simulink model "OfficalTeam58Code"  (R2023a)
settings: Solver=FixedStepAuto  StartTime=0.0  StopTime=inf  RelTol=1e-3  EnableMultiTasking=on
libraries: vexarmcortexlib x36, vexcommonlib x7, RoboticsPlayground x2
settings Model: Creator=arist  LastModifiedBy=arist
settings SolverCC: AutoInsertRateTranBlk=on
settings DataIOCC: LimitDataPoints=on  SignalLoggingSaveFormat=ModelDataLogs  ReturnWorkspaceOutputs=off
settings OptimizationCC: ExpressionDepthLimit=2147483647  LifeSpan=Inf  MaxStackSize=64  EfficientTunableParamExpr=on
settings DebuggingCC: UnderspecifiedInitializationDetection=Classic  MergeDetectMultiDrivingBlocksExec=none  InheritedTsInSrcMsg=none  MultiTaskRateTransMsg=warning  FcnCallInpInsideContextMsg=warning  StateNameClashWarn=warning  SFUnexpectedBacktrackingDiag=warning  SFNoUnconditionalDefaultTransitionDiag=warning  SFExecutionAtInitializationDiag=none  ArithmeticOperatorsInVariantConditions=warning
settings HardwareCC: ProdBitPerPointer=32  ProdBitPerSizeT=32  ProdBitPerPtrDiffT=32  ProdLargestAtomicInteger=Long  ProdLargestAtomicFloat=Double  ProdIntDivRoundTo=Undefined  ProdWordSize=32  ProdHWDeviceType=ARM Compatible->ARM Cortex
settings ModelReferenceCC: EnableRefExpFcnMdlSchedulingChecks=on  PropagateSignalLabelsOutOfModel=off
settings SFSimCC: MATLABDynamicMemAlloc=off  CustomCodeUndefinedFunction=UseInterfaceOnly
settings RTWCC: Description=Embedded Coder  SystemTargetFile=ert.tlc  HardwareBoard=ARM Cortex-based VEX Microcontroller  TemplateMakefile=ert_default_tmf  Toolchain=GNU Tools for VEX ARM Cortex
settings CodeAppCC: IgnoreCustomStorageClasses=off  CustomSymbolStrType=$N$R$M  StateflowObjectComments=on  InternalIdentifier=Classic
settings ERTTargetCC: CodeReplacementLibrary=GCC ARM Cortex-M3  MultiwordLength=2048  ConvertIfToSwitch=off  SuppressUnreachableDefaultCases=off

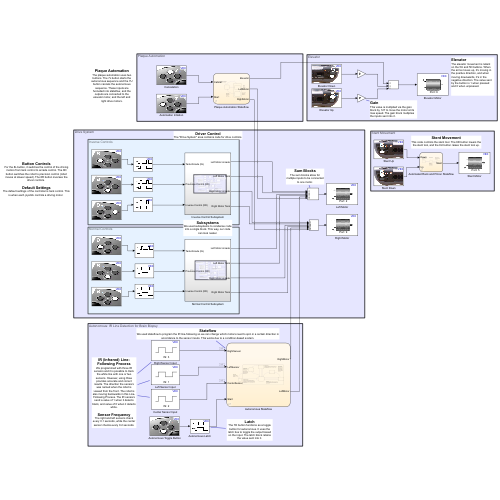
[thumbnail: Simulink's stored preview of the top-level diagram]
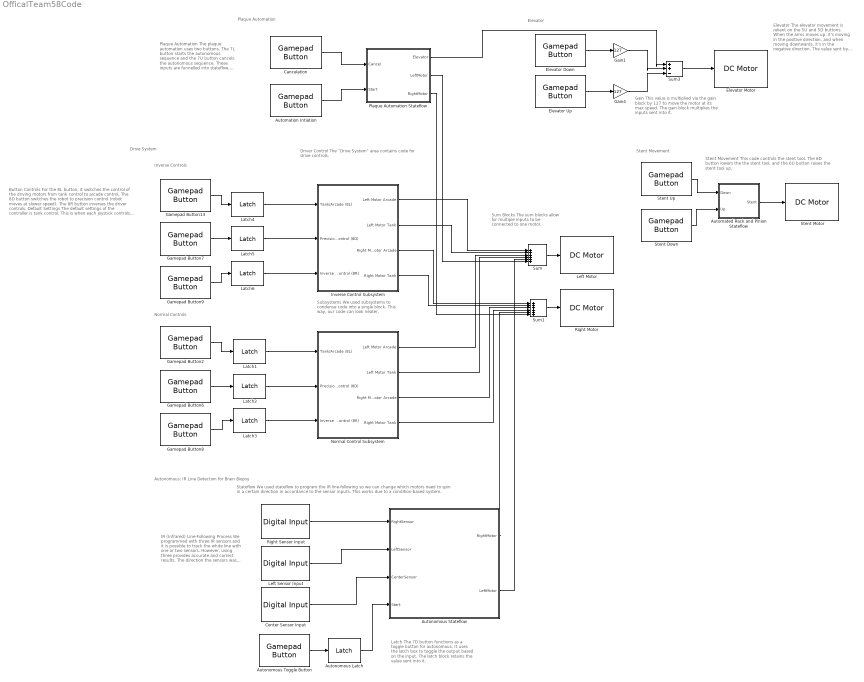
== system OfficalTeam58Code ==
  note: Driver Control
      | The "Drive System" area contains code for drive controls.
  note: Sum Blocks
      | The sum blocks allow for multiple inputs to be connected
      | to one motor.
  note: Subsystems
      | We used subsystems to condense code into a single block. This way, our code can look neater.
  note: Inverse Controls
  note: Autonomous: IR Line Detection for Brain Biopsy
  note: Drive System
  note: Normal Controls
  note: Plaque Automation
  note: Elevator
  note: Stent Movement
  note: Button Controls
      | For the 8L button, it switches the control of the driving motors from tank control to arcade control. The 8D button switches the robot to precision control (robot moves at slower speed). The 8R button inverses the driver controls.
      |
      | Default Settings
      | The default settings of the controller is tank control. This is when each joystick controls a driving motor.
  note: IR (Infrared) Line-Following Process
      | We programmed with three IR sensors and it is possible to track the white line with one or two sensors. However, using three provides accurate and correct results. The direction the sensors was named when the robot is viewed from the front. The robot is also moving backwards in this Line-Following Process. The IR sensors send a value of 1 when it detects black, and value of 0 when it detects white.
      |
      | Sensor Frequency
      | The right and left sensors check every 0.1 seconds, while the center sensor checks every 0.2 seconds.
  note: Latch
      | The 7D button functions as a toggle button for autonomous. It uses the latch box to toggle the output based on the input. The latch block retains the value sent into it.
  note: Stateflow
      | We used stateflow to program the IR line-following so we can change which motors need to spin in a certain direction in accordance to the sensor inputs. This works due to a condition-based system.
  note: Elevator
      | The elevator movement is reliant on the 5U and 5D buttons. When the arms moves up, it's moving in the positive direction, and when moving downwards, it's in the negative direction. The value sent by the button is 1 when pressed and 0 when unpressed.
  note: Plaque Automation
      | The plaque automation uses two buttons. The 7L button starts the autonomous sequence and the 7U button cancels the autonomous sequence. These inputs are funnelled into stateflow, and the outputs are connected to the elevator motor, and the left and right drive motors.
  note: Gain
      | This value is multiplied via the gain block by 127 to move the motor at its max speed. The gain block multiplies the inputs sent into it.
  note: Stent Movement
      | This code controls the stent tool. The 6D button lowers the the stent tool, and the 6U button raises the stent tool up.
  Automated Rack and Pinion Stateflow : Stateflow chart  AncestorBlock=RoboticsPlayground/Utilities and Hardware/Stateflow  TreatAsAtomicUnit=on
      settings: LibrarySourceBlock=RoboticsPlayground/Utilities and Hardware/Stateflow
  Automation Intiation : vexarmcortexlib/Gamepad/Gamepad Button  joystick=1  chan=7  button56=Down  button78=Left  SimulationIn=off  SampleTime=0.02
  Autonomous Latch : vexcommonlib/Latch  output0=off  BlockPlatform=vexv5
      settings: LibrarySourceBlock=vexv5lib/Utilities/Latch
  Autonomous Stateflow : Stateflow chart  AncestorBlock=RoboticsPlayground/Utilities and Hardware/Stateflow  TreatAsAtomicUnit=on
      settings: LibrarySourceBlock=RoboticsPlayground/Utilities and Hardware/Stateflow
  Autonomous Toggle Button : vexarmcortexlib/Gamepad/Gamepad Button  joystick=1  chan=7  button56=Up  button78=Down  SimulationIn=off  SampleTime=0.02
  Cancelation : vexarmcortexlib/Gamepad/Gamepad Button  joystick=1  chan=7  button56=Down  button78=Up  SimulationIn=off  SampleTime=0.02
  Center Sensor Input : vexarmcortexlib/Sensors/Digital Input  inChan=2  SimulationIn=off  SampleTime=0.2
  Elevator Down : vexarmcortexlib/Gamepad/Gamepad Button  joystick=1  chan=5  button56=Down  button78=Down  SimulationIn=off  SampleTime=0.02
  Elevator Motor : vexarmcortexlib/Actuators/DC Motor  motor=6  scaleFactor=1/13.5  SimulationOut=off
  Elevator Up : vexarmcortexlib/Gamepad/Gamepad Button  joystick=1  chan=5  button56=Up  button78=Down  SimulationIn=off  SampleTime=0.02
  Gain1 : Gain  Gain=127
  Gain4 : Gain  Gain=127
  Gamepad Button13 : vexarmcortexlib/Gamepad/Gamepad Button  joystick=1  chan=8  button56=Up  button78=Left  SimulationIn=off  SampleTime=0.02
  Gamepad Button2 : vexarmcortexlib/Gamepad/Gamepad Button  joystick=1  chan=8  button56=Up  button78=Left  SimulationIn=off  SampleTime=0.02
  Gamepad Button6 : vexarmcortexlib/Gamepad/Gamepad Button  joystick=1  chan=8  button56=Up  button78=Down  SimulationIn=off  SampleTime=0.02
  Gamepad Button7 : vexarmcortexlib/Gamepad/Gamepad Button  joystick=1  chan=8  button56=Up  button78=Down  SimulationIn=off  SampleTime=0.02
  Gamepad Button8 : vexarmcortexlib/Gamepad/Gamepad Button  joystick=1  chan=8  button56=Up  button78=Right  SimulationIn=off  SampleTime=0.02
  Gamepad Button9 : vexarmcortexlib/Gamepad/Gamepad Button  joystick=1  chan=8  button56=Up  button78=Right  SimulationIn=off  SampleTime=0.02
  Inverse Control Subsystem : Subsystem
  Latch{1..6} (6 alike) : vexcommonlib/Latch  output0=off  BlockPlatform=vexv5
      settings: LibrarySourceBlock=vexv5lib/Utilities/Latch
  Left Motor : vexarmcortexlib/Actuators/DC Motor  motor=2  scaleFactor=1/13.5  SimulationOut=off
  Left Sensor Input : vexarmcortexlib/Sensors/Digital Input  inChan=1  SimulationIn=off  SampleTime=0.1
  Normal Control Subsystem : Subsystem
  Plaque Automation Stateflow : Stateflow chart  AncestorBlock=RoboticsPlayground/Utilities and Hardware/Stateflow  TreatAsAtomicUnit=on
      settings: LibrarySourceBlock=RoboticsPlayground/Utilities and Hardware/Stateflow
  Right Motor : vexarmcortexlib/Actuators/DC Motor  motor=9  scaleFactor=1/13.5  SimulationOut=off
  Right Sensor Input : vexarmcortexlib/Sensors/Digital Input  inChan=3  SimulationIn=off  SampleTime=0.1
  Stent Down : vexarmcortexlib/Gamepad/Gamepad Button  joystick=1  chan=6  button56=Up  button78=Up  SimulationIn=off  SampleTime=0.02
  Stent Motor : vexarmcortexlib/Actuators/DC Motor  motor=5  scaleFactor=1/13.5  SimulationOut=off
  Stent Up : vexarmcortexlib/Gamepad/Gamepad Button  joystick=1  chan=6  button56=Down  button78=Left  SimulationIn=off  SampleTime=0.02
  Sum : Sum  Inputs=|++++++
  Sum1 : Sum  Inputs=|++++++
  Sum3 : Sum  Inputs=|++-
  wires:
  Gamepad Button2/1 -> Latch1/1
  Sum1/1 -> Right Motor/1
  Sum/1 -> Left Motor/1
  Autonomous Stateflow/1(RightMotor) -> Sum1/5
  Autonomous Stateflow/2(LeftMotor) -> Sum/5
  Autonomous Toggle Button/1 -> Autonomous Latch/1
  Center Sensor Input/1 -> Autonomous Stateflow/3(CenterSensor)
  Left Sensor Input/1 -> Autonomous Stateflow/2(LeftSensor)
  Right Sensor Input/1 -> Autonomous Stateflow/1(RightSensor)
  Gamepad Button6/1 -> Latch2/1
  Gamepad Button8/1 -> Latch3/1
  Latch1/1 -> Normal Control Subsystem/1(Tank/Arcade (8L))
  Latch2/1 -> Normal Control Subsystem/2(Precision Control (8D))
  Latch3/1 -> Normal Control Subsystem/3(Inverse Control (8R))
  Normal Control Subsystem/1(Left Motor Arcade) -> Sum/3
  Normal Control Subsystem/2(Left Motor Tank) -> Sum/4
  Normal Control Subsystem/3(Right Motor Arcade) -> Sum1/3
  Normal Control Subsystem/4(Right Motor Tank) -> Sum1/4
  Latch6/1 -> Inverse Control Subsystem/3(Inverse Control (8R))
  Latch5/1 -> Inverse Control Subsystem/2(Precision Control (8D))
  Gamepad Button9/1 -> Latch6/1
  Gamepad Button13/1 -> Latch4/1
  Gamepad Button7/1 -> Latch5/1
  Latch4/1 -> Inverse Control Subsystem/1(Tank/Arcade (8L))
  Inverse Control Subsystem/1(Left Motor Arcade) -> Sum/1
  Inverse Control Subsystem/2(Left Motor Tank) -> Sum/2
  Inverse Control Subsystem/4(Right Motor Tank) -> Sum1/2
  Inverse Control Subsystem/3(Right Motor Arcade) -> Sum1/1
  Autonomous Latch/1 -> Autonomous Stateflow/4(Start)
  Elevator Up/1 -> Gain4/1
  Plaque Automation Stateflow/2(LeftMotor) -> Sum/6
  Plaque Automation Stateflow/3(RightMotor) -> Sum1/6
  Gain1/1 -> Sum3/2
  Plaque Automation Stateflow/1(Elevator) -> Sum3/1
  Automation Intiation/1 -> Plaque Automation Stateflow/2(Start)
  Elevator Down/1 -> Gain1/1
  Cancelation/1 -> Plaque Automation Stateflow/1(Cancel)
  Sum3/1 -> Elevator Motor/1
  Gain4/1 -> Sum3/3
  Stent Up/1 -> Automated Rack and Pinion Stateflow/1(Down)
  Automated Rack and Pinion Stateflow/1(Stent) -> Stent Motor/1
  Stent Down/1 -> Automated Rack and Pinion Stateflow/2(Up)

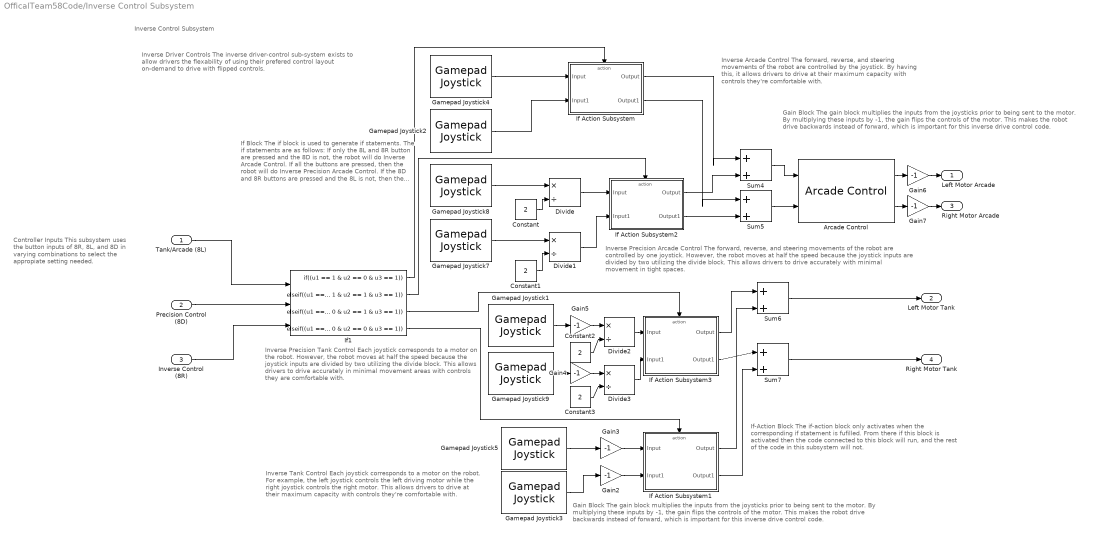
== system OfficalTeam58Code/Inverse Control Subsystem ==
  note: Inverse Driver Controls
      | The inverse driver-control sub-system exists to allow drivers
      | the flexability of using their prefered control layout on-demand to drive
      | with flipped controls.
  note: Inverse Control Subsystem
  note: If-Action Block
      | The if-action block only activates when the corresponding if statement is fufilled. From there if this block is activated then the code connected to this block will run, and the rest of the code in this subsystem will not.
  note: Controller Inputs
      | This subsystem uses the button inputs of 8R, 8L, and 8D
      | in varying combinations to select the appropiate setting needed.
  note: If Block
      | The if block is used to generate if statements. The if statements are as follows:
      | If only the 8L and 8R button are pressed and the 8D is not, the robot will do Inverse Arcade Control.
      | If all the buttons are pressed, then the robot will do Inverse Precision Arcade Control.
      | If the 8D and 8R buttons are pressed and the 8L is not, then the robot will do Inverse Precison Tank Control.
      | If only 8R is pressed and 8L and 8D are not, then the robot will do Inverse Tank Control.
  note: Inverse Precision Tank Control
      | Each joystick corresponds to a motor on the robot. However, the robot moves at half the speed because the joystick inputs are divided by two utilizing the divide block. This allows drivers to drive
      | accurately in minimal movement areas with controls they are
      | comfortable with.
  note: Inverse Tank Control
      | Each joystick corresponds to a motor on the robot. For example,
      | the left joystick controls the left driving motor while the right joystick
      | controls the right motor. This allows drivers to drive at their
      | maximum capacity with controls they're comfortable with.
  note: Inverse Precision Arcade Control
      | The forward, reverse, and steering movements of the robot are
      | controlled by one joystick. However, the robot moves at half the speed because the joystick inputs are divided by two utilizing the divide block. This allows drivers to drive accurately with minimal movement in tight spaces.
  note: Inverse Arcade Control
      | The forward, reverse, and steering movements of the robot are
      | controlled by the joystick. By having this, it allows drivers to
      | drive at their maximum capacity with controls they're comfortable
      | with.
  note: Gain Block
      | The gain block multiplies the inputs from the joysticks prior to being sent to the motor. By multiplying these inputs by -1, the gain flips the controls of the motor. This makes the robot drive backwards instead of forward, which is important for this inverse drive control code.
  note: Gain Block
      | The gain block multiplies the inputs from the joysticks prior to being sent to the motor. By multiplying these inputs by -1, the gain flips the controls of the motor. This makes the robot drive backwards instead of forward, which is important for this inverse drive control code.
  Tank/Arcade (8L) : Inport
  Precision Control (8D) : Inport  Port=2
  Inverse Control (8R) : Inport  Port=3
  Arcade Control : RoboticsPlayground/Utilities and Hardware/Arcade Control  SystemSampleTime=-1  VariantActivationTime=update diagram  Latency=0  AutoFrameSizeCalculation=off
      settings: SourceProductName=Robotics Playground
  Constant{,1..3} (4 alike) : Constant  Value=2
  Divide{,1..3} (4 alike) : Product  Inputs=*/
  Gain{2..7} (6 alike) : Gain  Gain=-1
  Gamepad Joystick{1,3..4,8} (4 alike) : vexarmcortexlib/Gamepad/Gamepad Joystick  joystick=1  chan=3  SimulationIn=off  SampleTime=0.02
  Gamepad Joystick2 : vexarmcortexlib/Gamepad/Gamepad Joystick  joystick=1  chan=4  SimulationIn=off  SampleTime=0.02
  Gamepad Joystick5 : vexarmcortexlib/Gamepad/Gamepad Joystick  joystick=1  chan=2  SimulationIn=off  SampleTime=0.02
  Gamepad Joystick7 : vexarmcortexlib/Gamepad/Gamepad Joystick  joystick=1  chan=4  SimulationIn=off  SampleTime=0.02
  Gamepad Joystick9 : vexarmcortexlib/Gamepad/Gamepad Joystick  joystick=1  chan=2  SimulationIn=off  SampleTime=0.02
  If Action Subsystem : Subsystem  TreatAsAtomicUnit=on
  If Action Subsystem1 : Subsystem  TreatAsAtomicUnit=on
  If Action Subsystem2 : Subsystem  TreatAsAtomicUnit=on
  If Action Subsystem3 : Subsystem  TreatAsAtomicUnit=on
  If1 : If  NumInputs=3  IfExpression=(u1 == 1 & u2 == 0 & u3 == 1)  ElseIfExpressions=(u1 == 1 & u2 == 1 & u3 == 1),(u1 == 0 & u2 == 1 & u3 == 1),(u1 == 0 & u2 == 0 & u3 == 1)  ShowElse=off
  Sum{4..7} (4 alike) : Sum  Inputs=|++
  Left Motor Arcade : Outport
  Left Motor Tank : Outport  Port=2
  Right Motor Arcade : Outport  Port=3
  Right Motor Tank : Outport  Port=4
  wires:
  Sum5/1 -> Arcade Control/2
  If1/4 -> If Action Subsystem1/Action
  If Action Subsystem1/1(Output) -> Sum6/2
  If1/3 -> If Action Subsystem3/Action
  If1/1 -> If Action Subsystem/Action
  If Action Subsystem2/1(Output) -> Sum4/2
  Divide2/1 -> If Action Subsystem3/1(Input)
  Constant1/1 -> Divide1/2
  If Action Subsystem1/2(Output1) -> Sum7/2
  Inverse Control (8R)/1 -> If1/3
  If Action Subsystem2/2(Output1) -> Sum5/2
  If Action Subsystem/2(Output1) -> Sum5/1
  Gamepad Joystick3/1 -> Gain2/1
  Sum6/1 -> Left Motor Tank/1
  If Action Subsystem/1(Output) -> Sum4/1
  Constant/1 -> Divide/2
  Divide1/1 -> If Action Subsystem2/2(Input1)
  If1/2 -> If Action Subsystem2/Action
  Divide3/1 -> If Action Subsystem3/2(Input1)
  Sum7/1 -> Right Motor Tank/1
  Constant3/1 -> Divide3/2
  Gamepad Joystick5/1 -> Gain3/1
  Sum4/1 -> Arcade Control/1
  Divide/1 -> If Action Subsystem2/1(Input)
  If Action Subsystem3/1(Output) -> Sum6/1
  Precision Control (8D)/1 -> If1/2
  Gamepad Joystick1/1 -> Gain5/1
  Gamepad Joystick9/1 -> Gain4/1
  Constant2/1 -> Divide2/2
  Arcade Control/1 -> Gain6/1
  If Action Subsystem3/2(Output1) -> Sum7/1
  Tank/Arcade (8L)/1 -> If1/1
  Arcade Control/2 -> Gain7/1
  Gamepad Joystick4/1 -> If Action Subsystem/1(Input)
  Gamepad Joystick8/1 -> Divide/1
  Gain2/1 -> If Action Subsystem1/2(Input1)
  Gain3/1 -> If Action Subsystem1/1(Input)
  Gain5/1 -> Divide2/1
  Gain4/1 -> Divide3/1
  Gamepad Joystick2/1 -> If Action Subsystem/2(Input1)
  Gamepad Joystick7/1 -> Divide1/1
  Gain6/1 -> Left Motor Arcade/1
  Gain7/1 -> Right Motor Arcade/1

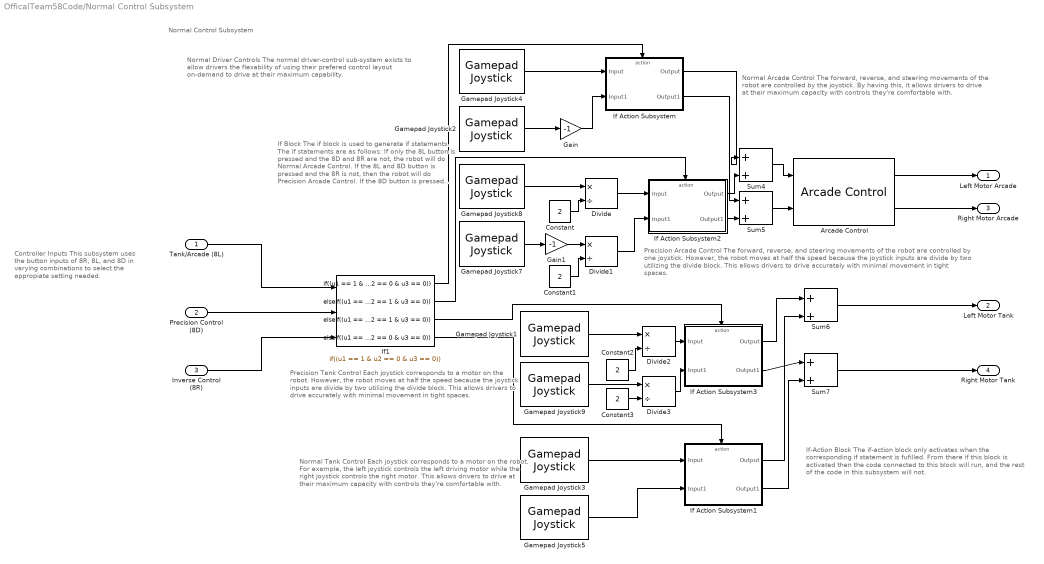
== system OfficalTeam58Code/Normal Control Subsystem ==
  note: If-Action Block
      | The if-action block only activates when the corresponding if statement is fufilled. From there if this block is activated then the code connected to this block will run, and the rest of the code in this subsystem will not.
  note: If Block
      | The if block is used to generate if statements. The if statements are as follows:
      | If only the 8L button is pressed and the 8D and 8R are not, the robot will do Normal Arcade Control.
      | If the 8L and 8D button is pressed and the 8R is not, then the robot will do Precision Arcade Control.
      | If the 8D button is pressed and the 8L and 8R are not, then the robot will do Precison Tank Control.
      | If none of the buttons are pressed, the robot will do Normal Tank Control.
  note: Precision Tank Control
      | Each joystick corresponds to a motor on the robot. However, the robot moves at half the speed because the joystick inputs are divide by two utilizing the divide block. This allows drivers to drive accurately with minimal movement in tight spaces.
  note: Normal Tank Control
      | Each joystick corresponds to a motor on the robot. For example,
      | the left joystick controls the left driving motor while the right joystick
      | controls the right motor. This allows drivers to drive at their
      | maximum capacity with controls they're comfortable with.
  note: Precision Arcade Control
      | The forward, reverse, and steering movements of the robot are
      | controlled by one joystick. However, the robot moves at half the speed because the joystick inputs are divide by two utilizing the divide block. This allows drivers to drive accurately with minimal movement in tight spaces.
  note: Normal Arcade Control
      | The forward, reverse, and steering movements of the robot are
      | controlled by the joystick. By having this, it allows drivers to
      | drive at their maximum capacity with controls they're comfortable with.
  note: Controller Inputs
      | This subsystem uses the button inputs of 8R, 8L, and 8D
      | in varying combinations to select the appropiate setting needed.
  note: Normal Driver Controls
      | The normal driver-control sub-system exists to allow drivers
      | the flexability of using their prefered control layout on-demand to
      | drive at their maximum capability.
  note: Normal Control Subsystem
  Tank/Arcade (8L) : Inport
  Precision Control (8D) : Inport  Port=2
  Inverse Control (8R) : Inport  Port=3
  Arcade Control : RoboticsPlayground/Utilities and Hardware/Arcade Control  SystemSampleTime=-1  VariantActivationTime=update diagram  Latency=0  AutoFrameSizeCalculation=off
      settings: SourceProductName=Robotics Playground
  Constant{,1..3} (4 alike) : Constant  Value=2
  Divide{,1..3} (4 alike) : Product  Inputs=*/
  Gain : Gain  Gain=-1
  Gain1 : Gain  Gain=-1
  Gamepad Joystick{1,3..4,8} (4 alike) : vexarmcortexlib/Gamepad/Gamepad Joystick  joystick=1  chan=3  SimulationIn=off  SampleTime=0.02
  Gamepad Joystick2 : vexarmcortexlib/Gamepad/Gamepad Joystick  joystick=1  chan=4  SimulationIn=off  SampleTime=0.02
  Gamepad Joystick5 : vexarmcortexlib/Gamepad/Gamepad Joystick  joystick=1  chan=2  SimulationIn=off  SampleTime=0.02
  Gamepad Joystick7 : vexarmcortexlib/Gamepad/Gamepad Joystick  joystick=1  chan=4  SimulationIn=off  SampleTime=0.02
  Gamepad Joystick9 : vexarmcortexlib/Gamepad/Gamepad Joystick  joystick=1  chan=2  SimulationIn=off  SampleTime=0.02
  If Action Subsystem : Subsystem  TreatAsAtomicUnit=on
  If Action Subsystem1 : Subsystem  TreatAsAtomicUnit=on
  If Action Subsystem2 : Subsystem  TreatAsAtomicUnit=on
  If Action Subsystem3 : Subsystem  TreatAsAtomicUnit=on
  If1 : If  NumInputs=3  IfExpression=(u1 == 1 & u2 == 0 & u3 == 0)  ElseIfExpressions=(u1 == 1 & u2 == 1 & u3 == 0),(u1 == 0 & u2 == 1 & u3 == 0),(u1 == 0 & u2 == 0 & u3 == 0)  ShowElse=off
  Sum{4..7} (4 alike) : Sum  Inputs=|++
  Left Motor Arcade : Outport
  Left Motor Tank : Outport  Port=2
  Right Motor Arcade : Outport  Port=3
  Right Motor Tank : Outport  Port=4
  wires:
  Sum5/1 -> Arcade Control/2
  If1/4 -> If Action Subsystem1/Action
  If Action Subsystem1/1(Output) -> Sum6/2
  If1/3 -> If Action Subsystem3/Action
  If1/1 -> If Action Subsystem/Action
  If Action Subsystem2/1(Output) -> Sum4/2
  Divide2/1 -> If Action Subsystem3/1(Input)
  Constant1/1 -> Divide1/2
  If Action Subsystem1/2(Output1) -> Sum7/2
  Inverse Control (8R)/1 -> If1/3
  If Action Subsystem2/2(Output1) -> Sum5/2
  Gain1/1 -> Divide1/1
  If Action Subsystem/2(Output1) -> Sum5/1
  Gamepad Joystick3/1 -> If Action Subsystem1/1(Input)
  Sum6/1 -> Left Motor Tank/1
  Gamepad Joystick2/1 -> Gain/1
  If Action Subsystem/1(Output) -> Sum4/1
  Constant/1 -> Divide/2
  Divide1/1 -> If Action Subsystem2/2(Input1)
  Gamepad Joystick8/1 -> Divide/1
  If1/2 -> If Action Subsystem2/Action
  Gamepad Joystick4/1 -> If Action Subsystem/1(Input)
  Gain/1 -> If Action Subsystem/2(Input1)
  Divide3/1 -> If Action Subsystem3/2(Input1)
  Gamepad Joystick7/1 -> Gain1/1
  Sum7/1 -> Right Motor Tank/1
  Constant3/1 -> Divide3/2
  Gamepad Joystick5/1 -> If Action Subsystem1/2(Input1)
  Sum4/1 -> Arcade Control/1
  Divide/1 -> If Action Subsystem2/1(Input)
  If Action Subsystem3/1(Output) -> Sum6/1
  Precision Control (8D)/1 -> If1/2
  Gamepad Joystick1/1 -> Divide2/1
  Gamepad Joystick9/1 -> Divide3/1
  Constant2/1 -> Divide2/2
  Arcade Control/1 -> Left Motor Arcade/1
  If Action Subsystem3/2(Output1) -> Sum7/1
  Tank/Arcade (8L)/1 -> If1/1
  Arcade Control/2 -> Right Motor Arcade/1

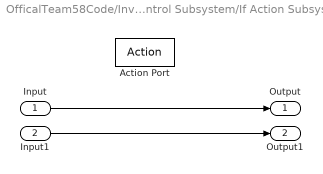
== system OfficalTeam58Code/Inverse Control Subsystem/If Action Subsystem ==
  Input : Inport
  Input1 : Inport  Port=2
  Action Port : ActionPort  ActionPortLabel=if((u1 == 1 & u2 == 0 & u3 == 1))
  Output : Outport
  Output1 : Outport  Port=2
  wires:
  Input/1 -> Output/1
  Input1/1 -> Output1/1

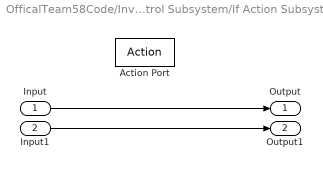
== system OfficalTeam58Code/Inverse Control Subsystem/If Action Subsystem1 ==
  Input : Inport
  Input1 : Inport  Port=2
  Action Port : ActionPort  ActionPortLabel=elseif((u1 == 0 & u2 == 0 & u3 == 1))
  Output : Outport
  Output1 : Outport  Port=2
  wires:
  Input/1 -> Output/1
  Input1/1 -> Output1/1

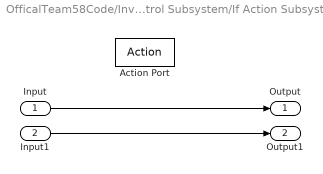
== system OfficalTeam58Code/Inverse Control Subsystem/If Action Subsystem2 ==
  Input : Inport
  Input1 : Inport  Port=2
  Action Port : ActionPort  ActionPortLabel=elseif((u1 == 1 & u2 == 1 & u3 == 1))
  Output : Outport
  Output1 : Outport  Port=2
  wires:
  Input/1 -> Output/1
  Input1/1 -> Output1/1

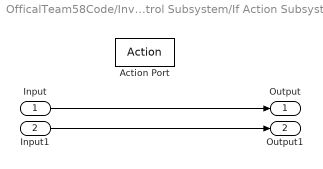
== system OfficalTeam58Code/Inverse Control Subsystem/If Action Subsystem3 ==
  Input : Inport
  Input1 : Inport  Port=2
  Action Port : ActionPort  ActionPortLabel=elseif((u1 == 0 & u2 == 1 & u3 == 1))
  Output : Outport
  Output1 : Outport  Port=2
  wires:
  Input/1 -> Output/1
  Input1/1 -> Output1/1

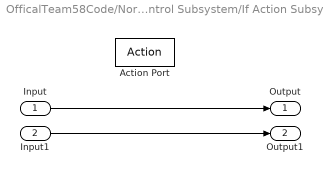
== system OfficalTeam58Code/Normal Control Subsystem/If Action Subsystem ==
  Input : Inport
  Input1 : Inport  Port=2
  Action Port : ActionPort  ActionPortLabel=if((u1 == 1 & u2 == 0 & u3 == 0))
  Output : Outport
  Output1 : Outport  Port=2
  wires:
  Input/1 -> Output/1
  Input1/1 -> Output1/1

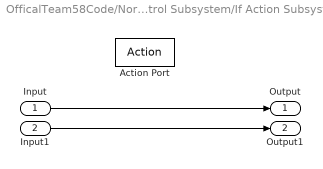
== system OfficalTeam58Code/Normal Control Subsystem/If Action Subsystem1 ==
  Input : Inport
  Input1 : Inport  Port=2
  Action Port : ActionPort  ActionPortLabel=elseif((u1 == 0 & u2 == 0 & u3 == 0))
  Output : Outport
  Output1 : Outport  Port=2
  wires:
  Input/1 -> Output/1
  Input1/1 -> Output1/1

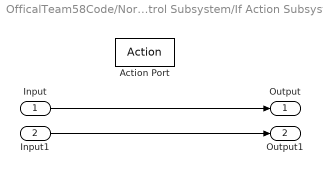
== system OfficalTeam58Code/Normal Control Subsystem/If Action Subsystem2 ==
  Input : Inport
  Input1 : Inport  Port=2
  Action Port : ActionPort  ActionPortLabel=elseif((u1 == 1 & u2 == 1 & u3 == 0))
  Output : Outport
  Output1 : Outport  Port=2
  wires:
  Input/1 -> Output/1
  Input1/1 -> Output1/1

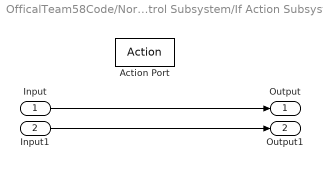
== system OfficalTeam58Code/Normal Control Subsystem/If Action Subsystem3 ==
  Input : Inport
  Input1 : Inport  Port=2
  Action Port : ActionPort  ActionPortLabel=elseif((u1 == 0 & u2 == 1 & u3 == 0))
  Output : Outport
  Output1 : Outport  Port=2
  wires:
  Input/1 -> Output/1
  Input1/1 -> Output1/1

== stateflow chart OfficalTeam58Code/Plaque Automation Stateflow ==
  note: Plaque Automation Sequence
      | .
  note: If the automation needs to stop at any point of the sequence, the 7U button can be pressed. This is done by encompassing the smaller states containing the autonomous in a super state.
  state Automation
    state Lower
      Elevator= 127;
    state StopandOut
      Elevator = 0;
      RightMotor = -70;
      LeftMotor = -70;
    Lower -> StopandOut : after(1.5,sec)
  state Start
    RightMotor=0;
    LeftMotor=0;
    Elevator=0;
  note: When the 7L button is pressed, the elevator will lower down at max speed.
  note: After 1.5 seconds, the elevator will stop, and the robot will move backwards.
  note: After 0.7 seconds, the robot will stop completely. This sequence will only repeat if the 7L button is pressed.
  Automation -> Start : [Cancel == 1]
  (default) -> Start
  Start -> Lower : [Start == 1]
  StopandOut -> Start : after(0.7,sec)
  data: Cancel input; Start input; Elevator output; LeftMotor output; RightMotor output

== stateflow chart OfficalTeam58Code/Autonomous Stateflow ==
  state IRAutonomous
    state RightTurn
      RightMotor = -43;
      LeftMotor = 43;
    note: Right Turning
        | If the left sensor detects white, then the robot will turn right until the left sensor detects black. Also, if the right sensor and center sensor detects black and the left sensor detects white, then the robot will also turn right.
    note: Faster Turning
        | After the robot has been turning for .4 seconds (400 milliseconds),
        | then the robot slightly speeds up its turn until the LeftSensor sees black.
        | This allows the robot to turn faster and either complete a sharp turn or get back on the track faster.
    state FasterRight
      RightMotor= -45;
      LeftMotor= 45;
    note: Faster Turning
        | After the robot has been turning for .4 seconds (400 milliseconds),
        | then the robot slightly speeds up its turn until the RightSensor sees black.
        | This allows the robot to turn faster and either complete a sharp turn or get back on the track faster.
    state FasterLeft
      RightMotor= 45;
      LeftMotor= -45;
    state StraightForward
      RightMotor=-55;
      LeftMotor=-57;
    state LeftTurn
      RightMotor = 43;
      LeftMotor = -43;
    note: Straight Forward
        | The robot will only start to go forward if the autonomous
        | toggle button (7D) is pressed and if the conditions are met.
        | The conditions required is that the left and right sensors need
        | to detect black while the center sensor needs to detect white.
        | Otherwise, it will make the needed adjustments based off the
        | conditions stated.
    note: Left Turning
        | If the right sensor detects white, then the robot will turn left until the right sensor detects black. Also, if the left sensor and center sensor detects black and the right sensor detects white, then the robot will also turn left.
    RightTurn -> FasterRight [order 2] : after(400,msec)
    StraightForward -> RightTurn [order 1] : [LeftSensor == 0]
    RightTurn -> StraightForward [order 1] : [LeftSensor == 1]
    StraightForward -> RightTurn [order 5] : [CenterSensor == 1 && RightSensor == 1 && LeftSensor == 0]
    FasterRight -> StraightForward : [LeftSensor == 1]
    FasterLeft -> StraightForward : [RightSensor == 1]
    LeftTurn -> FasterLeft [order 2] : after (400,msec)
    StraightForward -> LeftTurn [order 2] : [RightSensor == 0 && LeftSensor == 1 && CenterSensor == 1]
    StraightForward -> StraightForward [order 3] : [RightSensor == 1 && LeftSensor == 1 && CenterSensor == 0]
    LeftTurn -> StraightForward [order 1] : [RightSensor == 1]
    StraightForward -> LeftTurn [order 4] : [RightSensor == 0]
  note: "Autonomous" Superstate
      | Anytime the autonomous toggle (7D) is pressed during the
      | autonomous code, it stops.
  state Start
    RightMotor=0;
    LeftMotor=0;
  IRAutonomous -> Start : [Start == 0]
  (default) -> Start
  Start -> StraightForward : [Start == 1]
  data: RightMotor output; LeftMotor output; RightSensor input; LeftSensor input; CenterSensor input; Start input

== stateflow chart OfficalTeam58Code/Automated Rack and Pinion Stateflow ==
  note: When the 6D button is pressed, the stent arm is lowered. When the 6D button is released, the stent arm stays in position.
  note: When the 6U button is pressed, the stent arm is raised. When the 6D button is released, the stent arm stays in position.
  note: Stent Stateflow
  state Up
    Stent=45;
  state Start
    Stent=15;
  state Down
    Stent=-25;
  note: In order to prevent the tool from freely moving, power is continuously added to the motor when no buttons are pressed.
  (default) -> Start
  Start -> Up [order 2] : [Up == 1]
  Start -> Down [order 1] : [Down == 1]
  Up -> Start : [Up == 0]
  Down -> Start : [Down == 0]
  data: Down input; Stent output; Up input
